simulink model "framework"  (R2018b)
settings: Solver=FixedStepAuto  StartTime=0.0  StopTime=10.0  FixedStep=0.01  RelTol=1e-3
libraries: arduinolib x14, simulink x3
settings Model: SimulationMode=external  Creator=diktux  LastModifiedBy=diktux

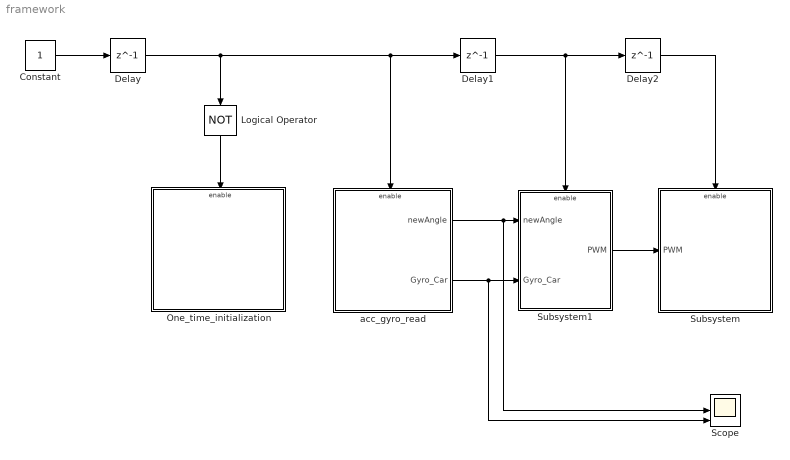
== system framework ==
  Constant : Constant
  Delay : Delay  DelayLength=1
  Delay1 : Delay  DelayLength=1
  Delay2 : Delay  DelayLength=1
  Logical Operator : Logic  Operator=NOT  AllPortsSameDT=off  OutDataTypeStr=boolean
  One_time_initialization : Subsystem
  Scope : Scope  NumInputPorts=3
  Subsystem : Subsystem
  Subsystem1 : Subsystem
  acc_gyro_read : Subsystem
  wires:
  Constant/1 -> Delay/1
  Delay/1 -> Logical Operator/1, acc_gyro_read/Enable, Delay1/1
  Logical Operator/1 -> One_time_initialization/Enable
  Delay1/1 -> Subsystem1/Enable, Delay2/1
  Delay2/1 -> Subsystem/Enable
  acc_gyro_read/2(Gyro_Car) -> Subsystem1/2(Gyro_Car), Scope/3
  acc_gyro_read/1(newAngle) -> Subsystem1/1(newAngle), Scope/2
  Subsystem1/1(PWM) -> Subsystem/1("PWM ")

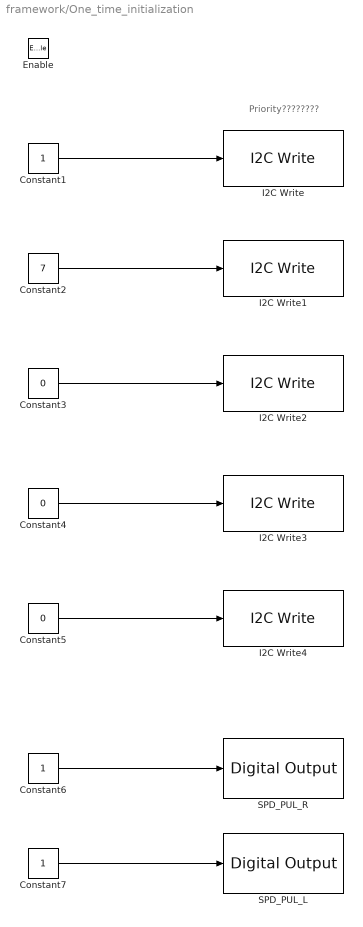
== system framework/One_time_initialization ==
  note: Priority????????
  Enable : EnablePort
  Constant1 : Constant
  Constant2 : Constant  Value=7
  Constant3 : Constant  Value=0
  Constant4 : Constant  Value=0
  Constant5 : Constant  Value=0
  Constant6 : Constant
  Constant7 : Constant
  I2C Write{,1..4} (5 alike) : arduinolib/I2C Write  I2CModule=0  Mode=Master  SlaveAddress=104  SlaveByteOrder=BigEndian  Direction=Transmitter  RegisterAddressMode=on  RegisterAddress=107  SlaveDataType=uint8  DataLength=1  NoAck=off  RepeatedStart=off  OutputStatus=off  blockPlatform=ARDUINO
      settings: SourceProductName=Simulink Support Package for Arduino Hardware  SourceProductBaseCode=ARDUINO
  SPD_PUL_L : arduinolib/Digital Output  pinNumber=9  blockPlatform=arduino
  SPD_PUL_R : arduinolib/Digital Output  pinNumber=12  blockPlatform=arduino
  wires:
  Constant4/1 -> I2C Write3/1
  Constant5/1 -> I2C Write4/1
  Constant2/1 -> I2C Write1/1
  Constant3/1 -> I2C Write2/1
  Constant1/1 -> I2C Write/1
  Constant7/1 -> SPD_PUL_L/1
  Constant6/1 -> SPD_PUL_R/1

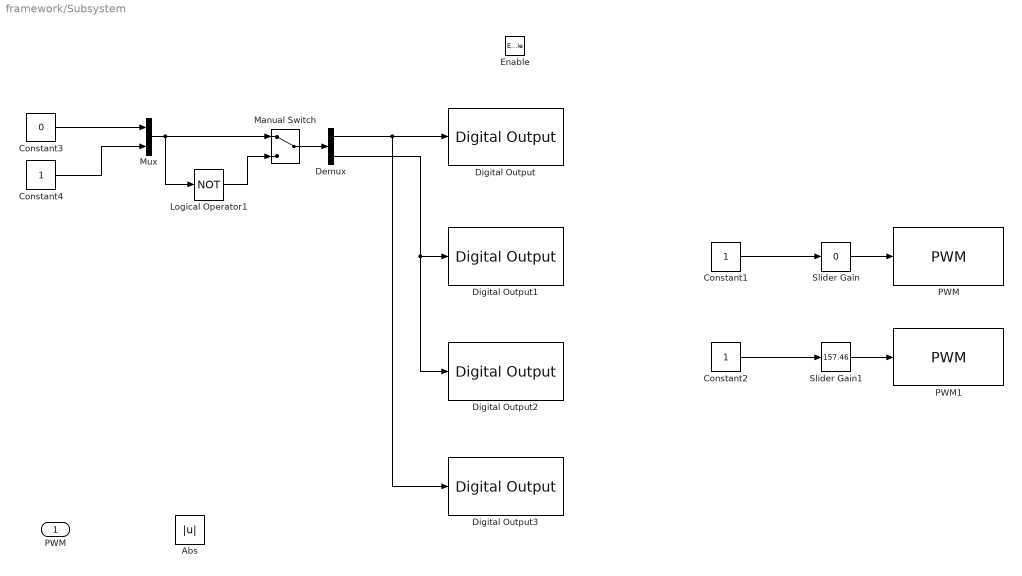
== system framework/Subsystem ==
  "PWM " : Inport
  Enable : EnablePort
  Abs : Abs
  Constant1 : Constant
  Constant2 : Constant
  Constant3 : Constant  Value=0
  Constant4 : Constant
  Demux : Demux  Outputs=2
  Digital Output : arduinolib/Digital Output  pinNumber=8  blockPlatform=arduino
  Digital Output1 : arduinolib/Digital Output  pinNumber=7  blockPlatform=arduino
  Digital Output2 : arduinolib/Digital Output  pinNumber=3  blockPlatform=arduino
  Digital Output3 : arduinolib/Digital Output  pinNumber=4  blockPlatform=arduino
  Logical Operator1 : Logic  Operator=NOT  AllPortsSameDT=off  OutDataTypeStr=boolean
  Manual Switch : ManualSwitch
  Mux : Mux  Inputs=2
  PWM : arduinolib/PWM  pinNumber=6  EnableInputFrequency=off  InitialFrequency=2000  InitialDutyCycle=0  NotificationType=None  blockPlatform=arduino
  PWM1 : arduinolib/PWM  pinNumber=5  EnableInputFrequency=off  InitialFrequency=2000  InitialDutyCycle=0  NotificationType=None  blockPlatform=arduino
  Slider Gain : simulink/Math Operations/Slider Gain  gain=0  low=0  high=255
  Slider Gain1 : simulink/Math Operations/Slider Gain  gain=157.46  low=0  high=255
  wires:
  Constant3/1 -> Mux/1
  Demux/1 -> Digital Output3/1, Digital Output/1
  Demux/2 -> Digital Output1/1, Digital Output2/1
  Logical Operator1/1 -> Manual Switch/2
  Slider Gain/1 -> PWM/1
  Constant1/1 -> Slider Gain/1
  Mux/1 -> Logical Operator1/1, Manual Switch/1
  Slider Gain1/1 -> PWM1/1
  Constant2/1 -> Slider Gain1/1
  Constant4/1 -> Mux/2
  Manual Switch/1 -> Demux/1

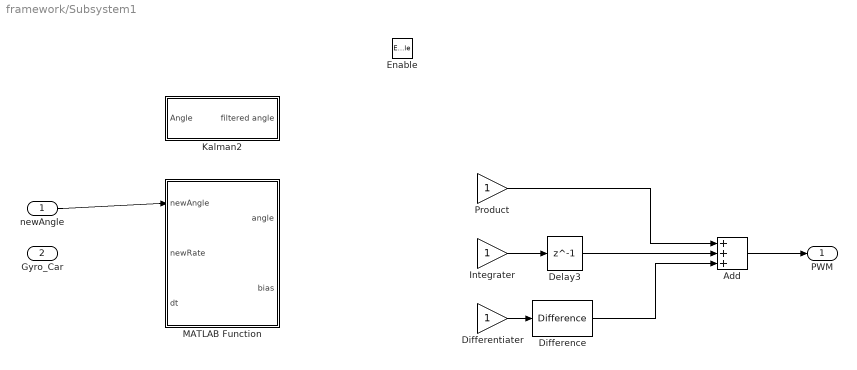
== system framework/Subsystem1 ==
  newAngle : Inport
  Gyro_Car : Inport  Port=2
  Enable : EnablePort
  Add : Sum  Inputs=3
  Delay3 : Delay  DelayLength=1
  Difference : simulink/Discrete/Difference  ICPrevInput=0.0  OutMin=[]  OutMax=[]  OutDataType=fixdt(1, 16)  OutScaling=2^-10  DoSatur=off
  Differentiater : Gain
  Integrater : Gain
  Kalman2 : Subsystem  mask{step_time=0.01}
      mask prompts: step_time "step time"
  MATLAB Function : MATLAB Function  TreatAsAtomicUnit=on
  Product : Gain
  PWM : Outport
  wires:
  Integrater/1 -> Delay3/1
  Differentiater/1 -> Difference/1
  ? -> Integrater/1, Differentiater/1, Product/1
  Delay3/1 -> Add/2
  Add/1 -> PWM/1
  Difference/1 -> Add/3
  Product/1 -> Add/1
  newAngle/1 -> MATLAB Function/1(newAngle)

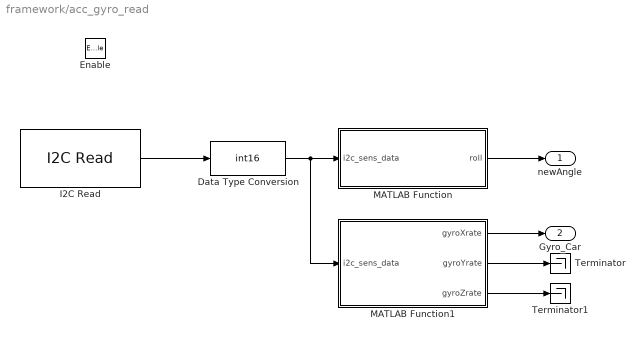
== system framework/acc_gyro_read ==
  Enable : EnablePort
  Data Type Conversion : DataTypeConversion  OutDataTypeStr=int16
  I2C Read : arduinolib/I2C Read  I2CModule=0  Mode=Master  SlaveAddress=104  SlaveByteOrder=BigEndian  Direction=Receiver  RegisterAddressMode=on  RegisterAddress=59  SlaveDataType=int16  DataLength=7  NoAck=off  RepeatedStart=off  OutputStatus=off  blockPlatform=ARDUINO  SampleTime=-1
      settings: SourceProductName=Simulink Support Package for Arduino Hardware  SourceProductBaseCode=ARDUINO
  MATLAB Function : MATLAB Function  TreatAsAtomicUnit=on
  MATLAB Function1 : MATLAB Function  TreatAsAtomicUnit=on
  Terminator : Terminator
  Terminator1 : Terminator
  newAngle : Outport
  Gyro_Car : Outport  Port=2
  wires:
  MATLAB Function1/2(gyroYrate) -> Terminator/1
  MATLAB Function1/1(gyroXrate) -> Gyro_Car/1
  MATLAB Function1/3(gyroZrate) -> Terminator1/1
  I2C Read/1 -> Data Type Conversion/1
  Data Type Conversion/1 -> MATLAB Function1/1(i2c_sens_data), MATLAB Function/1(i2c_sens_data)
  MATLAB Function/1(roll) -> newAngle/1

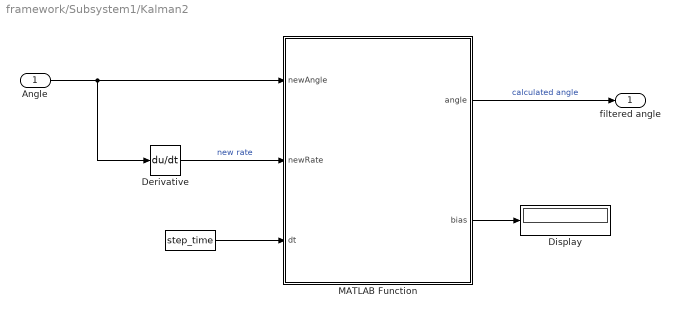
== system framework/Subsystem1/Kalman2 ==
  "Angle " : Inport
  "  " : Constant  Value=step_time  SampleTime=-1
  Derivative : Derivative  CoefficientInTFapproximation=-1
  Display : Display
  MATLAB Function : MATLAB Function  TreatAsAtomicUnit=on
  filtered angle : Outport
  wires:
  MATLAB Function/2(bias) -> Display/1
  "Angle "/1 -> MATLAB Function/1(newAngle), Derivative/1
  MATLAB Function/1(angle) -> filtered angle/1  "calculated angle"
  Derivative/1 -> MATLAB Function/2(newRate)  "new rate"
  "  "/1 -> MATLAB Function/3(dt)

== matlab function framework/acc_gyro_read/MATLAB Function1 ==
  data: i2c_sens_data input; gyroXrate output; gyroYrate output; gyroZrate output
function [gyroXrate,gyroYrate,gyroZrate] = fcn(i2c_sens_data)
gyroX = double(i2c_sens_data(5));
gyroY = double(i2c_sens_data(6));
gyroZ = double(i2c_sens_data(7));
gyroXrate = gyroX/131;
gyroYrate = gyroY/131;
gyroZrate = gyroZ/131;

== matlab function framework/acc_gyro_read/MATLAB Function ==
  data: i2c_sens_data input; roll output
function roll = fcn(i2c_sens_data)
accX = double(i2c_sens_data(1));
accY = double(i2c_sens_data(2));
accZ = double(i2c_sens_data(3));
roll = atan(accY / sqrt(accX * accX + accZ * accZ)) * 180/pi;

== matlab function framework/Subsystem1/MATLAB Function ==
  data: newAngle input; angle output; newRate input; dt input; bias output
function [angle,bias] = KalmanFil_Balanbot(newAngle,newRate,dt)
        % This script was adapted for its implementation in Simulink by R. Estrada (FH JOANNEUM 2017)
        % Based on KasBot V2  -  Kalman filter module - http:%www.x-firm.com/?page_id=145
        % Modified by Kristian Lauszus
        % More information: http:%blog.tkjelectronics.dk/2012/09/a-practical-approach-to-kalman-filter-and-how-to-implement-it

        % Discrete Kalman filter time update equations - Time Update ("Predict")
        % Update xhat - Project the state ahead
        
        coder.extrinsic('exist');
        
        % Declaration of persistent in memory variables (similar to declare global
        % variables)
   
        persistent init0 P K x;        
        
        % Initialization of typical sensor and noise variances 
        Q_angle = 0.001;
        Q_bias = 0.003; 
        R_measure = 0.03;
        
        % Declaration/initialization of main static matrices and vectors
        F = [1      -dt; 0      1];     % Transition matrix
        Q = [Q_angle  0; 0 Q_bias];     % Process noise covariance matrix  
        B = [dt ; 0];                   % Control-input model
        H = [1    0];                   % Observation model
        
        % SETUP: Executed only the first time      
        if isempty(init0)
            init0=0;
             % Declaration/initialization of main dynamic matrix and vectors
            P     = [0 0;0 0];  % Error covariance matrix
            K     = [0;0];      % Kalman gain vector
            x     = [0;0];      % State vector
        end

        % LOOP: Implementation of Kalman filter algorithm
        
        % Step 1 */          
        % Calculate prior state vector
        x = F * x + B * newRate;        

        % Step 2 */ 
        % Update estimation error covariance - Project the error covariance ahead               
         P = F * P * F' + Q * dt;  
                   
        % Step 3 */
        % Update estimate with measurement zk (newAngle)     
        y = newAngle - H * x;
        
        % Step 4 */
        % Discrete Kalman filter measurement update equations - Measurement Update ("Correct")              
        S = H * P * H' + R_measure;
        
        % Step 5 */
        % Compute the Kalman gain  
        K = P * H' / S;

        % Step 6 */
        % Update state vector
        x = x + K * y;
        
        % Step 7 */
        % Calculate estimation error covariance - Update the error covariance
        P = (eye(2) - K * H) * P;

        % RETURN: Update the function outputs
        angle = x(1);
        bias  = x(2);

== matlab function framework/Subsystem1/Kalman2/MATLAB Function ==
  settings: updateMethod=DISCRETE
  data: newAngle input; angle output; newRate input; dt input; bias output
function [angle,bias] = KalmanFil_Balanbot(newAngle,newRate,dt)
        % This script was adapted for its implementation in Simulink by R. Estrada (FH JOANNEUM 2017)
        % Based on KasBot V2  -  Kalman filter module - http:%www.x-firm.com/?page_id=145
        % Modified by Kristian Lauszus
        % More information: http:%blog.tkjelectronics.dk/2012/09/a-practical-approach-to-kalman-filter-and-how-to-implement-it

        % Discrete Kalman filter time update equations - Time Update ("Predict")
        % Update xhat - Project the state ahead
        
        coder.extrinsic('exist');
        
        % Declaration of persistent in memory variables (similar to declare global
        % variables)
   
        persistent init0 P K x;        
        
        % Initialization of typical sensor and noise variances 
        Q_angle = 0.001;
        Q_bias = 0.003; 
        R_measure = 0.03;
        
        % Declaration/initialization of main static matrices and vectors
        F = [1      -dt; 0      1];     % Transition matrix
        Q = [Q_angle  0; 0 Q_bias];     % Process noise covariance matrix  
        B = [dt ; 0];                   % Control-input model
        H = [1    0];                   % Observation model
        
        % SETUP: Executed only the first time      
        if isempty(init0)
            init0=0;
             % Declaration/initialization of main dynamic matrix and vectors
            P     = [0 0;0 0];  % Error covariance matrix
            K     = [0;0];      % Kalman gain vector
            x     = [0;0];      % State vector
        end

        % LOOP: Implementation of Kalman filter algorithm
        
        % Step 1 */          
        % Calculate prior state vector
        x = F * x + B * newRate;        

        % Step 2 */ 
        % Update estimation error covariance - Project the error covariance ahead               
         P = F * P * F' + Q * dt;  
                   
        % Step 3 */
        % Update estimate with measurement zk (newAngle)     
        y = newAngle - H * x;
        
        % Step 4 */
        % Discrete Kalman filter measurement update equations - Measurement Update ("Correct")              
        S = H * P * H' + R_measure;
        
        % Step 5 */
        % Compute the Kalman gain  
        K = P * H' / S;

        % Step 6 */
        % Update state vector
        x = x + K * y;
        
        % Step 7 */
        % Calculate estimation error covariance - Update the error covariance
        P = (eye(2) - K * H) * P;

        % RETURN: Update the function outputs
        angle = x(1);
        bias  = x(2);
